simulink library "gated_decay_choice"  (R2013a)
settings: Solver=ode45  StartTime=0.0  StopTime=10.0  RelTol=1e-3
undefined symbols (not defined in the file): alpha1, alpha2, beta
libraries: gated_decay_choice x1
settings Model: Creator=Leo  LastModifiedBy=Leo

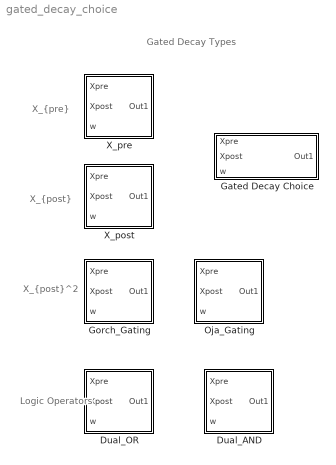
== system gated_decay_choice ==
  note: Logic
      | Operators
  note: X_{post}^2
  note: Gated Decay Types
  note: X_{post}
  note: X_{pre}
  Dual_AND : Subsystem
  Dual_OR : Subsystem
  Gated Decay Choice : Subsystem  BlockChoice=Gorch_Gating
      settings: TemplateBlock=self  MemberBlocks=Dual_AND,Dual_OR,Gorch_Gating,Oja_Gating,X_post,X_pre
  Gorch_Gating : Subsystem
  Oja_Gating : Subsystem
  X_post : Subsystem  AncestorBlock=gated_decay_choice/Gorch_Gating
  X_pre : Subsystem  AncestorBlock=gated_decay_choice/Gorch_Gating
  wires:
  ? -> ?
  ? -> ?

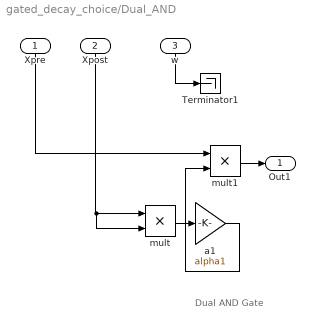
== system gated_decay_choice/Dual_AND ==
  note: Dual AND Gate
  Xpre : Inport
  Xpost : Inport  Port=2
  w : Inport  Port=3
  Terminator1 : Terminator
  a1 : Gain  Gain=alpha1
  mult : Product
  mult1 : Product
  Out1 : Outport
  wires:
  w/1 -> Terminator1/1
  Xpre/1 -> mult1/1
  Xpost/1 -> mult/1, mult/2
  mult/1 -> a1/1
  a1/1 -> mult1/2
  mult1/1 -> Out1/1

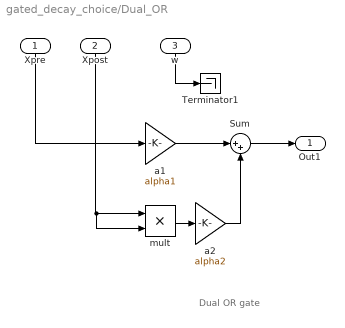
== system gated_decay_choice/Dual_OR ==
  note: Dual OR gate
  Xpre : Inport
  Xpost : Inport  Port=2
  w : Inport  Port=3
  Sum : Sum  Inputs=|++
  Terminator1 : Terminator
  a1 : Gain  Gain=alpha1
  a2 : Gain  Gain=alpha2
  mult : Product
  Out1 : Outport
  wires:
  mult/1 -> a2/1
  Xpost/1 -> mult/2, mult/1
  Xpre/1 -> a1/1
  w/1 -> Terminator1/1
  a2/1 -> Sum/2
  a1/1 -> Sum/1
  Sum/1 -> Out1/1

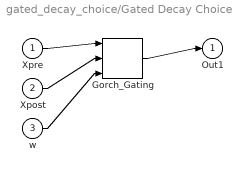
== system gated_decay_choice/Gated Decay Choice ==
  Xpre : Inport
  Xpost : Inport  Port=2
  w : Inport  Port=3
  Gorch_Gating : gated_decay_choice/Gorch_Gating
  Out1 : Outport
  wires:
  Xpre/1 -> Gorch_Gating/1
  Xpost/1 -> Gorch_Gating/2
  w/1 -> Gorch_Gating/3
  Gorch_Gating/1 -> Out1/1

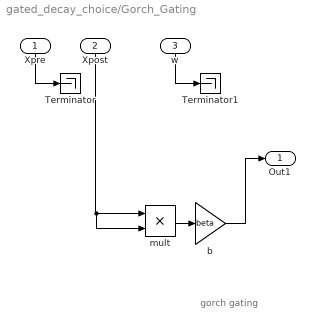
== system gated_decay_choice/Gorch_Gating ==
  note: gorch gating
  Xpre : Inport
  Xpost : Inport  Port=2
  w : Inport  Port=3
  Terminator : Terminator
  Terminator1 : Terminator
  b : Gain  Gain=beta
  mult : Product
  Out1 : Outport
  wires:
  w/1 -> Terminator1/1
  Xpre/1 -> Terminator/1
  Xpost/1 -> mult/1, mult/2
  b/1 -> Out1/1
  mult/1 -> b/1

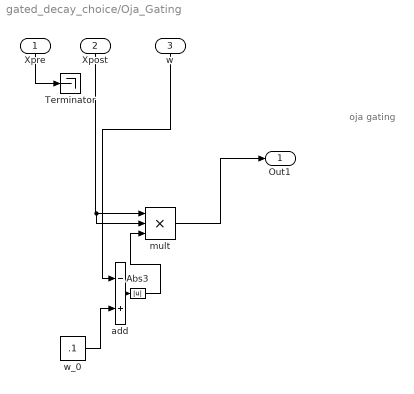
== system gated_decay_choice/Oja_Gating ==
  note: oja gating
  Xpre : Inport
  Xpost : Inport  Port=2
  w : Inport  Port=3
  Abs3 : Abs
  Terminator : Terminator
  add : Sum  Inputs=-+
  mult : Product  Inputs=3
  w_0 : Constant  Value=.1
  Out1 : Outport
  wires:
  Abs3/1 -> mult/3
  w/1 -> add/1
  add/1 -> Abs3/1
  w_0/1 -> add/2
  mult/1 -> Out1/1
  Xpost/1 -> mult/2, mult/1
  Xpre/1 -> Terminator/1

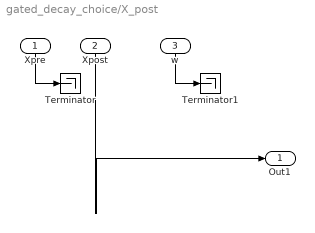
== system gated_decay_choice/X_post ==
  Xpre : Inport
  Xpost : Inport  Port=2
  w : Inport  Port=3
  Terminator : Terminator
  Terminator1 : Terminator
  Out1 : Outport
  wires:
  Xpost/1 -> Out1/1
  Xpre/1 -> Terminator/1
  w/1 -> Terminator1/1

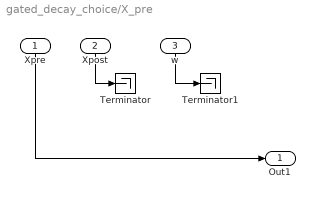
== system gated_decay_choice/X_pre ==
  Xpre : Inport
  Xpost : Inport  Port=2
  w : Inport  Port=3
  Terminator : Terminator
  Terminator1 : Terminator
  Out1 : Outport
  wires:
  w/1 -> Terminator1/1
  Xpre/1 -> Out1/1
  Xpost/1 -> Terminator/1
